simulink model "sim_vdp_delta"  (R2016a)
settings: Solver=VariableStepAuto  StartTime=0.0  StopTime=50  RelTol=1e-3
values from neighbouring files (symbols this model uses):
  delta = 10    [plot_reachsets.m]    (also in plot_roa.m = 5)
  x0 = [x01; x02; x03]    [plot_reachsets.m]    (also in plot_roa.m = x02)
libraries: simulink x3
settings Model: Creator=y977li  LastModifiedBy=y977li
settings DataIOCC: InitialState=x0  SaveFormat=Array  SaveState=on

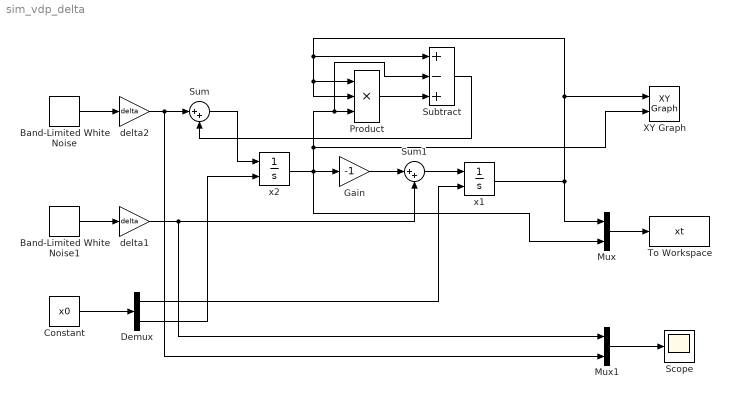
== system sim_vdp_delta ==
  Band-Limited White Noise : simulink/Sources/Band-Limited White Noise  Cov=[0.001]  Ts=0.01  seed=seed
  Band-Limited White Noise1 : simulink/Sources/Band-Limited White Noise  Cov=[0.001]  Ts=0.01  seed=seed
  Constant : Constant  Value=x0
  Demux : Demux  Outputs=2
  Gain : Gain  Gain=-1
  Mux : Mux  Inputs=2
  Mux1 : Mux  Inputs=2
  Product : Product  Inputs=3
  Scope : Scope
  Subtract : Sum  Inputs=+-+
  Sum : Sum  Inputs=|++
  Sum1 : Sum  Inputs=|++
  To Workspace : ToWorkspace  VariableName=xt  SampleTime=-1
  XY Graph : simulink/Sinks/XY Graph  xmin=-3  xmax=3  ymin=-3  ymax=3  st=-1
  delta1 : Gain  Gain=delta
  delta2 : Gain  Gain=delta
  x1 : Integrator  InitialConditionSource=external  InitialCondition=0.9  ContinuousStateAttributes='x1'
  x2 : Integrator  InitialConditionSource=external  ContinuousStateAttributes='x2'
  wires:
  x2/1 -> Mux/2, XY Graph/2, Subtract/2, Product/3, Gain/1
  x1/1 -> XY Graph/1, Product/2, Product/1, Subtract/1, Mux/1
  Product/1 -> Subtract/3
  Band-Limited White Noise/1 -> delta2/1
  delta2/1 -> Mux1/2, Sum/1
  Subtract/1 -> Sum/2
  Sum/1 -> x2/1
  Band-Limited White Noise1/1 -> delta1/1
  Gain/1 -> Sum1/1
  Sum1/1 -> x1/1
  delta1/1 -> Mux1/1, Sum1/2
  Mux/1 -> To Workspace/1
  Constant/1 -> Demux/1
  Demux/1 -> x1/2
  Demux/2 -> x2/2
  Mux1/1 -> Scope/1
